simulink model "comp"  (Simulink 4.0)
settings: Solver=ode23  StartTime=0.0  StopTime=22  RelTol=1e-3
values from neighbouring files (symbols this model uses):
  x0 = [2;0]    [linid.m]    (also in nonlinid.m = [0;0]; sfdcmotorin.m = []; sfdcmotorout.m = [])
undefined symbols (not defined in the file or in its folder): u0
libraries: cstblocks x1
settings Model: LastModifiedBy=R.Babuska

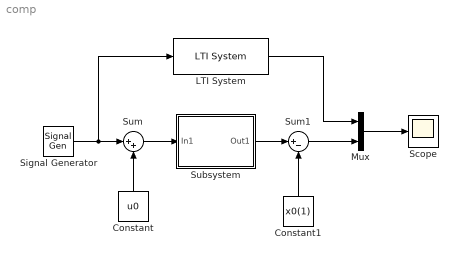
== system comp ==
  Constant : Constant  Orientation=up  Value=u0
  Constant1 : Constant  Orientation=up  Value=x0(1)
  LTI System : cstblocks/LTI System  sys=G  IC=0
  Mux : Mux  Inputs=2
  Scope : Scope
      settings: TimeRange=25  YMin=-0.03  YMax=0.03  SaveToWorkspace=off  SaveName=ScopeData  LimitDataPoints=on  MaxDataPoints=5000
  Signal Generator : SignalGenerator  WaveForm=square  Amplitude=.1  Frequency=1/10  Units=Hertz
  Subsystem : Subsystem  SimViewingDevice=off
      settings: Permissions=ReadWrite  RTWFcnNameOpts=Auto  RTWFileNameOpts=Auto
  Sum : Sum  Inputs=|++  SaturateOnIntegerOverflow=on
  Sum1 : Sum  Inputs=|+-  SaturateOnIntegerOverflow=on
  wires:
  Signal Generator/1 -> Sum/1, LTI System/1
  Sum/1 -> Subsystem/1(In1)
  Constant/1 -> Sum/2
  Constant1/1 -> Sum1/2
  Mux/1 -> Scope/1
  Subsystem/1(Out1) -> Sum1/1
  Sum1/1 -> Mux/2
  LTI System/1 -> Mux/1

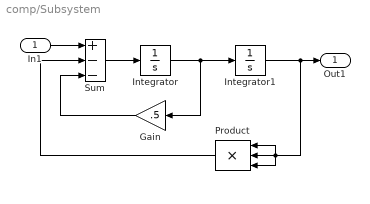
== system comp/Subsystem ==
  In1 : Inport  Port=1  PortDimensions=-1  SampleTime=-1  DataType=auto
      settings: SignalType=auto
  Gain : Gain  Orientation=left  Gain=.5  Multiplication=Element-wise(K.*u)  SaturateOnIntegerOverflow=on
  Integrator : Integrator  ExternalReset=none  InitialConditionSource=internal  InitialCondition=x0(2)  LimitOutput=off  UpperSaturationLimit=inf  LowerSaturationLimit=-inf  ShowSaturationPort=off  ShowStatePort=off  AbsoluteTolerance=auto
  Integrator1 : Integrator  ExternalReset=none  InitialConditionSource=internal  InitialCondition=x0(1)  LimitOutput=off  UpperSaturationLimit=inf  LowerSaturationLimit=-inf  ShowSaturationPort=off  ShowStatePort=off  AbsoluteTolerance=auto
  Product : Product  Orientation=left  Inputs=3  Multiplication=Element-wise(.*)  SaturateOnIntegerOverflow=on
  Sum : Sum  Inputs=+--  SaturateOnIntegerOverflow=on
  Out1 : Outport  Port=1
  wires:
  Integrator/1 -> Integrator1/1, Gain/1
  Sum/1 -> Integrator/1
  Integrator1/1 -> Product/2, Product/1, Product/3, Out1/1
  Product/1 -> Sum/2
  Gain/1 -> Sum/3
  In1/1 -> Sum/1
